simulink model "tasks"  (R2018a)
settings: Solver=VariableStepAuto  StartTime=0.0  StopTime=10.0  RelTol=1e-3
settings Model: EnablePacing=on  Creator=U500304  LastModifiedBy=U500304

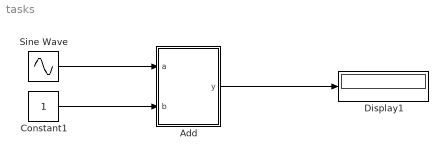
== system tasks ==
  Add : MATLAB Function  TreatAsAtomicUnit=on
  Constant1 : Constant
  Display1 : Display
  Sine Wave : Sin  Amplitude=10  SampleTime=0
  wires:
  Sine Wave/1 -> Add/1(a)
  Constant1/1 -> Add/2(b)
  Add/1(y) -> Display1/1

== matlab function tasks/Add ==
  data: y output; a input; b input
function y = callfoo(a, b)
y = 0.0;
coder.updateBuildInfo('addSourceFiles','matlab.c');
coder.cinclude('matlab.h');
y = coder.ceval('add', a, b);
end
